simulink model "PARTE1_YHOLI"  (R2025b)
settings: Solver=VariableStepAuto  StartTime=0.0  StopTime=160  RelTol=1e-3
libraries: cstblocks x2, simulink x2, slpidlib x1
settings Model: Creator=yholi  LastModifiedBy=yholi

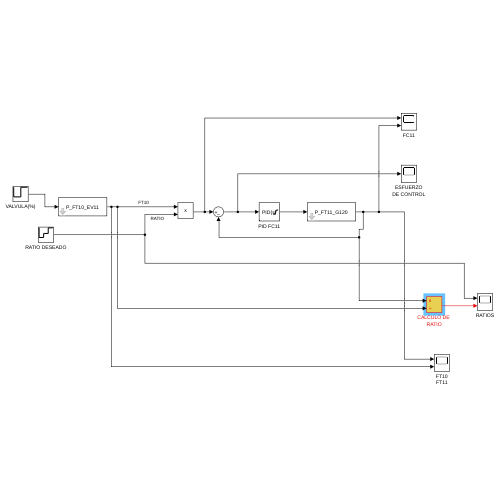
[thumbnail: Simulink's stored preview of the top-level diagram]
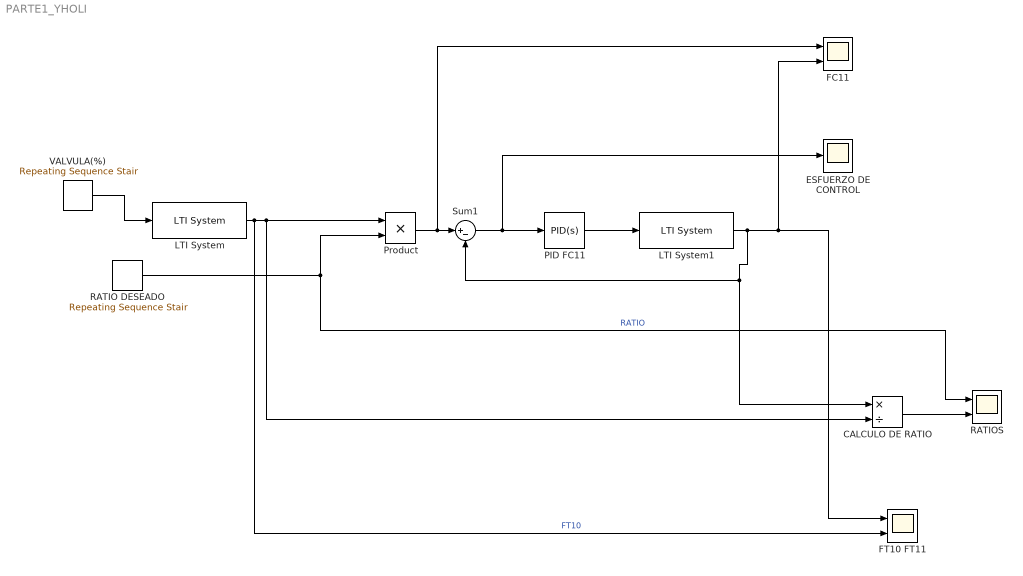
== system PARTE1_YHOLI ==
  CALCULO DE RATIO : Product  Inputs=*/
  ESFUERZO DE CONTROL : Scope
      settings: ActiveDisplayYMinimum=-23.559549317642759  ActiveDisplayYMaximum=22.419853836652408
  FC11 : Scope  NumInputPorts=2
      settings: ActiveDisplayYMinimum=-27.230453750734043  ActiveDisplayYMaximum=105.88693523331035
  FT10 FT11 : Scope  NumInputPorts=2
      settings: ActiveDisplayYMinimum=-12.113883907662448  ActiveDisplayYMaximum=102.37061841712799  DataLoggingVariableName=ScopeData3
  LTI System : cstblocks/LTI System  sys=P_FT10_EV11  IC=[]  PadeOrder=0
  LTI System1 : cstblocks/LTI System  sys=P_FT11_G120  IC=[]  PadeOrder=0
  PID FC11 : slpidlib/PID Controller  Controller=PID  Form=Parallel  TimeDomain=Continuous-time  UseExternalTs=off  SampleTime=-1  IntegratorMethod=Forward Euler  FilterMethod=Forward Euler  ControllerParametersSource=internal  P=2.4859  I=3.6647  UseKiTs=off  D=0.051352  UseExternalDerivativeSource=off  N=100  UseFilter=on  TunerSelectOption=Transfer Function Based (PID Tuner App)  InitialConditionSource=internal  InitialConditionForIntegrator=0  InitialConditionForFilter=0  DifferentiatorICPrevScaledInput=0  ExternalReset=none  TrackingMode=off  Kt=1  LimitOutput=on  SatLimitsSource=internal  UpperSaturationLimit=100  LowerSaturationLimit=0  LinearizeAsGain=on  AntiWindupMode=none  Kb=1  LimitIntegrator=off  UpperIntegratorSaturationLimit=inf  LowerIntegratorSaturationLimit=-inf  POutMin=[]  POutMax=[]  IOutMin=[]  IOutMax=[]  DOutMin=[]  DOutMax=[]  NOutMin=[]  NOutMax=[]  SumOutMin=[]  SumOutMax=[]  SaturationOutMin=[]  SaturationOutMax=[]  PParamMin=[]  PParamMax=[]  IParamMin=[]  IParamMax=[]  DParamMin=[]  DParamMax=[]  NParamMin=[]  NParamMax=[]  KbParamMin=[]  KbParamMax=[]  KtParamMin=[]  KtParamMax=[]  KbOutMin=[]  KbOutMax=[]  KtOutMin=[]  KtOutMax=[]  IntegratorOutMin=[]  IntegratorOutMax=[]  FilterOutMin=[]  FilterOutMax=[]  SumI1OutMin=[]  SumI1OutMax=[]  SumI2OutMin=[]  SumI2OutMax=[]  SumI3OutMin=[]  SumI3OutMax=[]  SumI4OutMin=[]  SumI4OutMax=[]  SumDOutMin=[]  SumDOutMax=[]  DifferentiatorOutMin=[]  DifferentiatorOutMax=[]  FilterDiffOutCoefMin=[]  FilterDiffOutCoefMax=[]  ReciprocalOutMin=[]  ReciprocalOutMax=[]  SumDenOutMin=[]  SumDenOutMax=[]  SumNumOutMin=[]  SumNumOutMax=[]  DivideOutMin=[]  DivideOutMax=[]  UdiffTsProdOutMin=[]  UdiffTsProdOutMax=[]  NTsProdOutMin=[]  NTsProdOutMax=[]  UintegralTsProdOutMin=[]  UintegralTsProdOutMax=[]  UngainTsProdOutMin=[]  UngainTsProdOutMax=[]  ClampingZeroOutDataTypeStr=Inherit: Inherit via back propagation  ClampingZeroOutMin=[]  ClampingZeroOutMax=[]  FilterDenConstantOutDataTypeStr=Inherit: Inherit via back propagation  FilterDenConstantOutMin=[]  FilterDenConstantOutMax=[]  PCopyOutDataTypeStr=Inherit: Inherit via back propagation  PCopyOutMin=[]  PCopyOutMax=[]  NCopyOutDataTypeStr=Inherit: Inherit via back propagation  NCopyOutMin=[]  NCopyOutMax=[]  IntegratorContinuousStateAttributes=''  IntegratorStateMustResolveToSignalObject=off  IntegratorRTWStateStorageClass=Auto  FilterContinuousStateAttributes=''  FilterStateMustResolveToSignalObject=off  FilterRTWStateStorageClass=Auto  ParallelPVariant=InternalParameters  IdealPVariant=Disabled  IVariant=InternalParameters  DVariant=InternalParameters  IntegratorVariant=Continuous  SatVariant=Enabled  AWVariant=Passthrough  PCopyVariant=Disabled  TRVariant=Disabled  FdbkBlocksVariant=Forward  IdealPFdbkVariant=Disabled  SatFdbkVariant=Disabled  DerivativeFilterVariant=ContFilter  NVariant=InternalParameters  NCopyVariant=Disabled  FilterICVariant=InternalICsFilter  IntegratorICVariant=InternalICs  ExternalResetVariant=Disabled  TRSumVariant=Passthrough  SumFdbkVariant=Disabled  SumVariant=Sum_PID  TsampFilterVariant=InternalTs  TsampNgainVariant=Passthrough  TsampIntegralVariant=Disabled_SignalSpec  ExternalSaturationOutDataTypeStr=Inherit: Same as second input  DerivativeSourceVariant=ErrorSignal  PreIntVariant=InternalPreInt
  Product : Product
  RATIO DESEADO : simulink/Sources/Repeating Sequence Stair  OutValues=[1 1.2 1.5].'  tsamp=40  OutMin=[]  OutMax=[]  OutDataTypeStr=double  OutputDataTypeScalingMode=double  OutDataType=fixdt(0,8)  ConRadixGroup=Best Precision: Vector-wise  OutScaling=2^-12
  RATIOS : Scope  NumInputPorts=2
      settings: ActiveDisplayYMinimum=-2.43031779149576  ActiveDisplayYMaximum=4.0672580742961406  DataLoggingVariableName=ScopeData2
  Sum1 : Sum  Inputs=|+-
  VALVULA(%) : simulink/Sources/Repeating Sequence Stair  OutValues=[20 50].'  tsamp=40  OutMin=[]  OutMax=[]  OutDataTypeStr=double  OutputDataTypeScalingMode=double  OutDataType=fixdt(0,8)  ConRadixGroup=Best Precision: Vector-wise  OutScaling=2^-12
  wires:
  VALVULA(%)/1 -> LTI System/1
  PID FC11/1 -> LTI System1/1
  LTI System/1 -> FT10 FT11/2, CALCULO DE RATIO/2, Product/1  "FT10"
  LTI System1/1 -> Sum1/2, CALCULO DE RATIO/1, FC11/2, FT10 FT11/1
  CALCULO DE RATIO/1 -> RATIOS/2
  RATIO DESEADO/1 -> RATIOS/1, Product/2  "RATIO"
  Sum1/1 -> ESFUERZO DE CONTROL/1, PID FC11/1
  Product/1 -> FC11/1, Sum1/1
